simulink model "Motor_position"  (R2020a)
settings: Solver=ode23s  StartTime=0.0  StopTime=0.1  MaxStep=0.001  RelTol=1e-3
values from neighbouring files (symbols this model uses):
  b = 3.5077E-6    [Ques_4_Parameters.sldd]
  J = 3.2284E-6    [Ques_4_Parameters.sldd]
  K = 0.0274    [Ques_4_Parameters.sldd]
  kd = 0.5    [Ques_4_Parameters.sldd]
  ki = 4810.0    [Ques_4_Parameters.sldd]
  kp = 98.0    [Ques_4_Parameters.sldd]
  L = 2.75E-6    [Ques_4_Parameters.sldd]
  n = 119828.0    [Ques_4_Parameters.sldd]
  R = 4.0    [Ques_4_Parameters.sldd]
settings Model: DataDictionary=Ques_4_Parameters.sldd  Creator=DELL  LastModifiedBy=DELL

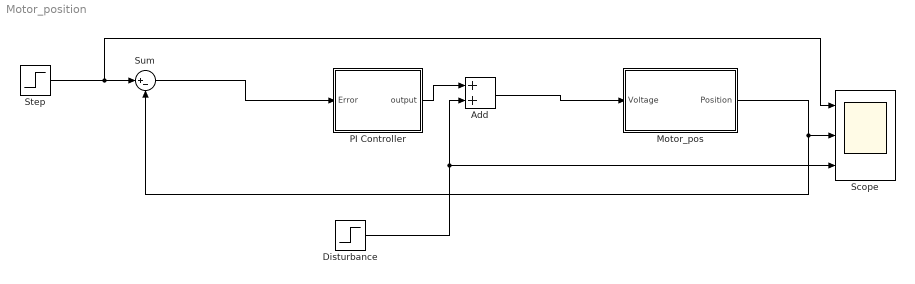
== system Motor_position ==
  Add : Sum
  Disturbance : Step  Time=0.06  SampleTime=0
  Motor_pos : Subsystem
  PI Controller : Subsystem
  Scope : Scope  NumInputPorts=3
  Step : Step  Time=0  SampleTime=0
  Sum : Sum  Inputs=|+-
  wires:
  Motor_pos/1(Position) -> Sum/2, Scope/2
  Step/1 -> Scope/1, Sum/1
  PI Controller/1(output) -> Add/1
  Add/1 -> Motor_pos/1(Voltage)
  Sum/1 -> PI Controller/1(Error)
  Disturbance/1 -> Scope/3, Add/2

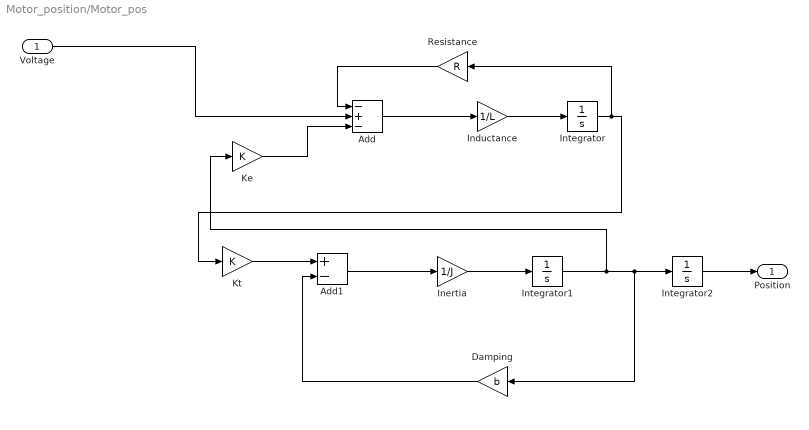
== system Motor_position/Motor_pos ==
  Voltage : Inport
  Add : Sum  Inputs=-+-
  Add1 : Sum  Inputs=+-
  Damping : Gain  Gain=b
  Inductance : Gain  Gain=1/L
  Inertia : Gain  Gain=1/J
  Integrator : Integrator
  Integrator1 : Integrator
  Integrator2 : Integrator
  Ke : Gain  Gain=K
  Kt : Gain  Gain=K
  Resistance : Gain  Gain=R
  Position : Outport
  wires:
  Add1/1 -> Inertia/1
  Kt/1 -> Add1/1
  Add/1 -> Inductance/1
  Ke/1 -> Add/3
  Inductance/1 -> Integrator/1
  Integrator/1 -> Resistance/1, Kt/1
  Integrator1/1 -> Ke/1, Damping/1, Integrator2/1
  Inertia/1 -> Integrator1/1
  Resistance/1 -> Add/1
  Integrator2/1 -> Position/1
  Voltage/1 -> Add/2
  Damping/1 -> Add1/2

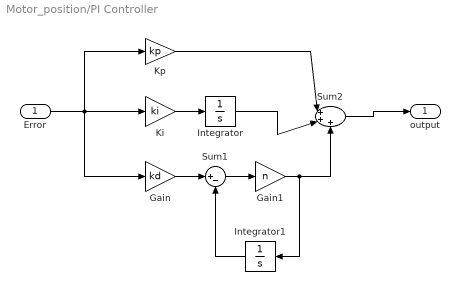
== system Motor_position/PI Controller ==
  Error : Inport
  Gain : Gain  Gain=kd
  Gain1 : Gain  Gain=n
  Integrator : Integrator
  Integrator1 : Integrator
  Ki : Gain  Gain=ki
  Kp : Gain  Gain=kp
  Sum1 : Sum  Inputs=|+-
  Sum2 : Sum  Inputs=|+++
  output : Outport
  wires:
  Kp/1 -> Sum2/1
  Sum2/1 -> output/1
  Ki/1 -> Integrator/1
  Sum1/1 -> Gain1/1
  Gain1/1 -> Integrator1/1, Sum2/3
  Error/1 -> Gain/1, Ki/1, Kp/1
  Integrator/1 -> Sum2/2
  Integrator1/1 -> Sum1/2
  Gain/1 -> Sum1/1
